simulink model "accumulator_basic_ok"  (R2019b)
settings: Solver=ode4  StartTime=0.0  StopTime=100  FixedStep=0.001  RelTol=1e-3
values from neighbouring files (symbols this model uses):
  Am = 7.2    [value.m]
  Aw = 3.812*10^(-12)    (= 3.812e-12)    [value.m]
  valve_radius = 0.01    [value.m]
undefined symbols (not defined in the file or in its folder): sigbuilder_block
libraries: fl_lib x11, nesl_utility x8, sh_lib x5
settings Model: Creator=remil  LastModifiedBy=remil
settings SimscapeCC: SimscapeLogType=all  SimscapeLogSimulationStatistics=on  SimscapeLogOpenViewer=on

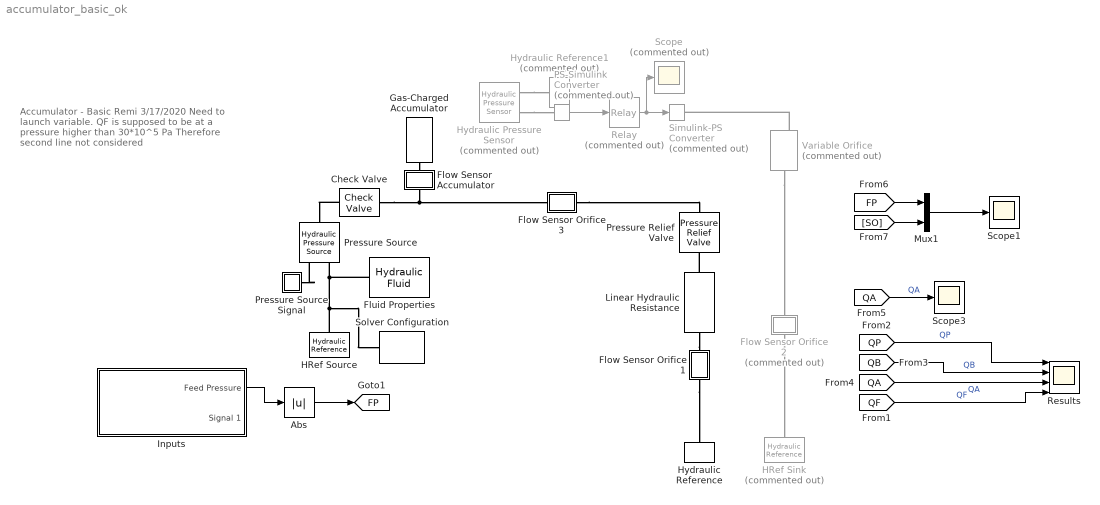
== system accumulator_basic_ok ==
  note: Accumulator - Basic
      | Remi 3/17/2020
      | Need to launch variable.
      | QF is supposed to be at a pressure
      | higher than 30*10^5 Pa Therefore
      | second line not considered
  Abs : Abs
  Check Valve : sh_lib/Valves/Directional Valves/Check Valve  Tag=Factory Generic  area_max=pi*(valve_radius)^2 m^2  pres_crack=30000 Pa  pres_max=120000 Pa  C_d=0.7  A_leak=1e-12 m^2  lam_spec=1  B_lam=0.999  Re_cr=12  dynamic=1  tau=0.1 s  area_init=1e-12 m^2
      settings: SourceProductName=Simscape Fluids  SourceProductBaseCode=SH  InternalSimscapePortConfiguration="{\"Bottom\":[],\"Left\":[{\"id\":\"A\",\"label\":\"A\",\"type\":\"foundation.hydraulic.hydraulic\"}],\"Right\":[{\"id\":\"B\",\"label\":\"B\",\"type\":\"foundation.hydraulic.hydraulic\"}],\"Top\":[]}"
  Flow Sensor Accumulator : Subsystem
      mask Display: disp('QA')
  Flow Sensor Orifice 1 : Subsystem
      mask Display: disp('QP');
  Flow Sensor Orifice 2 : Subsystem  Commented=on
      mask Display: disp('QB');
  Flow Sensor Orifice 3 : Subsystem
      mask Display: disp('QF');
  Fluid Properties : sh_lib/Hydraulic Utilities/Hydraulic Fluid  DataSource=1  SelFluid=1  SysTemp=60  TrapAir=0.005  ViscDerFactor=1  range_error=2
      settings: SourceProductName=Simscape Fluids
  Gas-Charged Accumulator : sh_lib/Accumulators/Gas-Charged Accumulator  capacity=2.5 gal  dead_volume=0.08 l  pr_preload=30e5 Pa  k_sh=1.4  stiff_coeff=1e12 Pa/m^3  penetr_coeff=1e10 s*Pa/m^6  flow_rate_specify=off  flow_rate_priority=High  flow_rate=0.005 m^3/s  flow_rate_nominal_specify=off  flow_rate_nominal_unit=m^3/s  flow_rate_nominal_value=1  liquid_volume_specify=on  liquid_volume_priority=High  liquid_volume=0 gal  liquid_volume_nominal_specify=off  liquid_volume_nominal_unit=m^3  liquid_volume_nominal_value=1  liquid_pressure_specify=off  liquid_pressure_priority=None  liquid_pressure=1.01325e+5 Pa  liquid_pressure_nominal_specify=off  liquid_pressure_nominal_unit=Pa  liquid_pressure_nominal_value=1
      settings: SourceProductName=Simscape Fluids  SourceProductBaseCode=SH  InternalSimscapePortConfiguration="{\"Bottom\":[],\"Left\":[],\"Right\":[{\"id\":\"A\",\"label\":\"A\",\"type\":\"foundation.hydraulic.hydraulic\"}],\"Top\":[]}"
  HRef Sink : fl_lib/Hydraulic/Hydraulic Elements/Hydraulic Reference  Tag=Factory Generic  Commented=on
      settings: SourceProductName=Simscape
  HRef Source : fl_lib/Hydraulic/Hydraulic Elements/Hydraulic Reference  Tag=Factory Generic
      settings: SourceProductName=Simscape
  Hydraulic Pressure Sensor : fl_lib/Hydraulic/Hydraulic Sensors/Hydraulic Pressure Sensor  Commented=on
      settings: SourceProductName=Simscape
  Hydraulic Reference : fl_lib/Hydraulic/Hydraulic Elements/Hydraulic Reference
      settings: SourceProductName=Simscape
  Hydraulic Reference1 : fl_lib/Hydraulic/Hydraulic Elements/Hydraulic Reference  Commented=on
      settings: SourceProductName=Simscape
  "Inputs " : Subsystem  Tag=STV Subsys  LoadFcn=sigbuilder_block('load');  StartFcn=sigbuilder_block('start');  StopFcn=sigbuilder_block('stop');  ClipboardFcn=sigbuilder_block('clipboard');  mask(Sigbuilder block){tuvar=[0:10]}
      mask help: Sigbuilder GUI
      mask init:
      | if ~strcmp(get_param(bdroot(gcbh),'SimulationStatus'),'stopped') tuvar = sigbuilder_block('maskInit'); end
      settings: CopyFcn=sigbuilder_block('copy');  DeleteFcn=sigbuilder_block('delete');  ModelCloseFcn=sigbuilder_block('modelClose');  PreSaveFcn=sigbuilder_block('preSave');  PauseFcn=sigbuilder_block('pause')  ContinueFcn=sigbuilder_block('continue')  NameChangeFcn=sigbuilder_block('namechange');  OpenFcn=sigbuilder_block('open',[6 30 1428 681.75 ]);  CloseFcn=sigbuilder_block('close');
      mask Display: plot(0, 0, 100, 100,[2, 2, 32, 32, 2], [68, 8, 8, 68, 68],[32, 2], [38, 38], [32, 19, 2],[53, 60, 44], [32, 17, 17, 2],[16, 16, 31, 31]);txt = getActiveGroup(gcbh);text(2, 100, txt,'verticalAlignment', 'top');
  Linear Hydraulic Resistance : fl_lib/Hydraulic/Hydraulic Elements/Linear Hydraulic Resistance  resistance=1/(Am*Aw) Pa/(m^3/s)  q_specify=off  q_priority=None  q=0.001 m^3/s  q_nominal_specify=off  q_nominal_unit=m^3/s  q_nominal_value=1  p_specify=off  p_priority=None  p=0 Pa  p_nominal_specify=off  p_nominal_unit=Pa  p_nominal_value=1
      settings: SourceProductName=Simscape  SourceProductBaseCode=SS  InternalSimscapePortConfiguration="{\"Bottom\":[],\"Left\":[{\"id\":\"A\",\"label\":\"A\",\"type\":\"foundation.hydraulic.hydraulic\"}],\"Right\":[{\"id\":\"B\",\"label\":\"B\",\"type\":\"foundation.hydraulic.hydraulic\"}],\"Top\":[]}"
  Mux1 : Mux  Inputs=2
      settings: DisplayOption=signals
  PS-Simulink Converter : nesl_utility/PS-Simulink Converter  Commented=on  PhysicalDomain=network_engine_domain  SubClassName=ps_output  LeftPortType=input  RightPortType=output  PseudoPeriodic=off  Frequencies=[]  Unit=inherit  AffineConversion=off
  Pressure Source : fl_lib/Hydraulic/Hydraulic Sources/Hydraulic Pressure Source  Tag=Factory Generic
      settings: SourceProductName=Simscape  SourceProductBaseCode=SS  InternalSimscapePortConfiguration="{\"Bottom\":[],\"Left\":[{\"id\":\"P\",\"label\":\"P\",\"type\":\"foundation.hydraulic.hydraulic\"}],\"Right\":[{\"id\":\"S\",\"label\":\"S\",\"type\":\"input\"},{\"id\":\"T\",\"label\":\"T\",\"type\":\"foundation.hydraulic.hydraulic\"}],\"Top\":[]}"
  Pressure Source Signal : Subsystem
      mask Display: disp('FP')
  Pressure Relief Valve : sh_lib/Valves/Pressure Control Valves/Pressure Relief Valve  valve_area_spec=1  p_diff_TLU=[30.15e5 : 15e3 : 31.35e5] Pa  area_TLU=[1 : 1 : 9] .* 1e-5 m^2  area_max=pi*(valve_radius)^2 m^2  pres_set=30e5 Pa  reg_range=5e5 Pa  C_d=0.7  A_leak=1e-12 m^2  lam_spec=1  B_lam=0.999  Re_cr=12  dynamic=0  tau=0.1 s  area_init=1e-12 m^2
      settings: SourceProductName=Simscape Fluids  SourceProductBaseCode=SH  InternalSimscapePortConfiguration="{\"Bottom\":[],\"Left\":[{\"id\":\"A\",\"label\":\"A\",\"type\":\"foundation.hydraulic.hydraulic\"}],\"Right\":[{\"id\":\"B\",\"label\":\"B\",\"type\":\"foundation.hydraulic.hydraulic\"}],\"Top\":[]}"
  Relay : Relay  Commented=on  OnSwitchValue=30*10^5  OffSwitchValue=30*10^5  OnOutputValue=0  OffOutputValue=0.01
  Results : Scope  NumInputPorts=4
  Scope : Scope  Commented=on
  Scope1 : Scope
  Scope3 : Scope
  Simulink-PS Converter : nesl_utility/Simulink-PS Converter  Commented=on  PhysicalDomain=network_engine_domain  SubClassName=ps_input  LeftPortType=input  RightPortType=output  PseudoPeriodic=off  Frequencies=[]  NoiseDistribution=none  NoiseParameters=[]  Unit=1  AffineConversion=off  FilteringAndDerivatives=filter  SimscapeFilterOrder=1  InputFilterTimeConstant=0.001  UdotUserProvided=0
  Solver Configuration : nesl_utility/Solver Configuration  PhysicalDomain=network_engine_domain  SubClassName=solver  LeftPortType=input  RightPortType=generic  Tones=[]  Harmonics=[]  SimulateNoise=off  Profile=off  UseLocalSampling=off  EnableSwitchedLinearOptims=on  FrequencyDomain=off  UseCCode=off  RelTol=0.001  AbsTol=1e-06  MinStep=1e-09  ToWorkspace=off  RevertToSquareIcSolve=off  NumHomotopyIterations=100  PhasorMode=off  PhasorModeNumHarmonics=1  DoDC=on  ResidualTolerance=1e-9  UseLocalSolver=on  LocalSolverChoice=NE_BACKWARD_EULER_ADVANCER  LocalSolverSampleTime=.001  DoFixedCost=on  MaxNonlinIter=3  MaxModeIter=2  LinearAlgebra=auto  EquationFormulation=NE_TIME_EF  DelaysMemoryBudget=1024  AutomaticFiltering=on  FilteringTimeConstant=0.001  PartitionStorageMethod=AS_NEEDED  PartitionMemoryBudget=1024  PartitionMethod=FAST
  Variable Orifice : sh_lib/Orifices/Variable Orifice  Commented=on  mdl_type=1  area_max=pi*(valve_radius)^2 m^2  opening_max=2*0.01 m  opening_tab=[-.002, 0, .002, .005, .015] m  area_tab=[1e-09, 2.0352e-07, 4.0736e-05, .00011438, .00034356] m^2  pressure_tab=[-10000000, -5000000, -2000000, 2000000, 5000000, 10000000] Pa  flow_rate_tab=[-1e-07, -7.0711e-08, -4.4721e-08, 4.4721e-08, 7.0711e-08, 1e-07; -2.0352e-05, -1.4391e-05, -9.1017e-06, 9.1017e-06, 1.4391e-05, 2.0352e-05; -.0040736, -.0028805, -.0018218, .0018218, .0028805, .0040736; -.011438, -.0080879, -.0051152, .0051152, .0080879, .011438; -.034356, -.024293, -.015364, .015364, .024293, .034356] m^3/s  interp_method=1  extrap_method=1  or=1  C_d=0.7  x_0=0 m  A_leak=1e-12 m^2  lam_spec=1  B_lam=0.999  Re_cr=12  flow_rate_specify=on  flow_rate_priority=High  flow_rate=0 m^3/s  flow_rate_nominal_specify=off  flow_rate_nominal_unit=m^3/s  flow_rate_nominal_value=1  pressure_drop_specify=off  pressure_drop_priority=None  pressure_drop=0 Pa  pressure_drop_nominal_specify=off  pressure_drop_nominal_unit=Pa  pressure_drop_nominal_value=1
      settings: SourceProductName=Simscape Fluids  SourceProductBaseCode=SH  InternalSimscapePortConfiguration="{\"Bottom\":[],\"Left\":[{\"id\":\"S\",\"label\":\"S\",\"type\":\"input\"},{\"id\":\"A\",\"label\":\"A\",\"type\":\"foundation.hydraulic.hydraulic\"}],\"Right\":[{\"id\":\"B\",\"label\":\"B\",\"type\":\"foundation.hydraulic.hydraulic\"}],\"Top\":[]}"
  tag scope: FP=global
  wires:
  Abs/1 -> [FP]
  [QP] -> Results/1  "QP"
  [QB] -> Results/2  "QB"
  [QA] -> Results/3  "QA"
  [QA] -> Scope3/1  "QA"
  PS-Simulink Converter/1 -> Relay/1
  Relay/1 -> Scope/1, Simulink-PS Converter/1
  Mux1/1 -> Scope1/1
  [FP] -> Mux1/1
  [SO] -> Mux1/2
  [QF] -> Results/4  "QF"
  "Inputs "/1(Feed Pressure) -> Abs/1
  connections:
  Flow Sensor Orifice 2/LConn1 -- HRef Sink/LConn1
  Pressure Source/RConn2 -- Solver Configuration/RConn1 -- HRef Source/LConn1 -- Fluid Properties/RConn1
  Gas-Charged Accumulator/RConn1 -- Flow Sensor Accumulator/RConn1
  Pressure Source Signal/RConn1 -- Pressure Source/RConn1
  Variable Orifice/LConn1 -- Simulink-PS Converter/RConn1
  Flow Sensor Orifice 3/RConn1 -- Pressure Relief Valve/LConn1
  Check Valve/RConn1 -- Flow Sensor Accumulator/LConn1 -- Flow Sensor Orifice 3/LConn1
  Hydraulic Pressure Sensor/RConn2 -- PS-Simulink Converter/LConn1
  Hydraulic Pressure Sensor/RConn1 -- Hydraulic Reference1/LConn1
  Linear Hydraulic Resistance/RConn1 -- Flow Sensor Orifice 1/LConn1
  Flow Sensor Orifice 1/RConn1 -- Hydraulic Reference/LConn1
  Check Valve/LConn1 -- Pressure Source/LConn1
  Linear Hydraulic Resistance/LConn1 -- Pressure Relief Valve/RConn1
  Variable Orifice/RConn1 -- Flow Sensor Orifice 2/RConn1

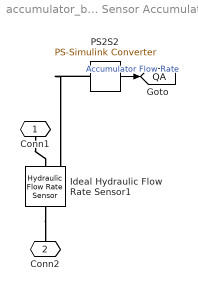
== system accumulator_basic_ok/Flow Sensor Accumulator ==
  Ideal Hydraulic Flow Rate Sensor1 : fl_lib/Hydraulic/Hydraulic Sensors/Hydraulic Flow Rate Sensor  Tag=Factory Generic
      settings: SourceProductName=Simscape
  PS2S2 : nesl_utility/PS-Simulink Converter  PhysicalDomain=network_engine_domain  SubClassName=ps_output  LeftPortType=input  RightPortType=output  PseudoPeriodic=off  Frequencies=[]  Unit=1  AffineConversion=off
  Conn1 : PMIOPort  Side=Right
  Conn2 : PMIOPort  Port=2  Side=Left
  tag scope: QA=global
  wires:
  PS2S2/1 -> [QA]  "Accumulator Flow Rate"
  connections:
  PS2S2/LConn1 -- Ideal Hydraulic Flow Rate Sensor1/RConn1
  Conn1/RConn1 -- Ideal Hydraulic Flow Rate Sensor1/RConn2
  Ideal Hydraulic Flow Rate Sensor1/LConn1 -- Conn2/RConn1

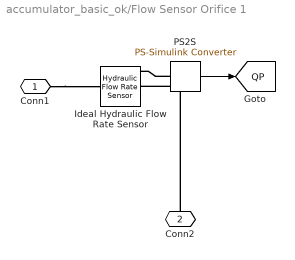
== system accumulator_basic_ok/Flow Sensor Orifice 1 ==
  Ideal Hydraulic Flow Rate Sensor : fl_lib/Hydraulic/Hydraulic Sensors/Hydraulic Flow Rate Sensor  Tag=Factory Generic
      settings: SourceProductName=Simscape
  PS2S : nesl_utility/PS-Simulink Converter  PhysicalDomain=network_engine_domain  SubClassName=ps_output  LeftPortType=input  RightPortType=output  PseudoPeriodic=off  Frequencies=[]  Unit=1  AffineConversion=off
  Conn1 : PMIOPort  Side=Left
  Conn2 : PMIOPort  Port=2  Side=Right
  tag scope: QP=global
  wires:
  PS2S/1 -> [QP]
  connections:
  PS2S/LConn1 -- Ideal Hydraulic Flow Rate Sensor/RConn1
  Conn2/RConn1 -- Ideal Hydraulic Flow Rate Sensor/RConn2
  Conn1/RConn1 -- Ideal Hydraulic Flow Rate Sensor/LConn1

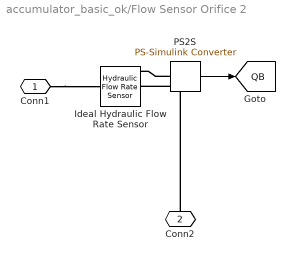
== system accumulator_basic_ok/Flow Sensor Orifice 2 ==
  Ideal Hydraulic Flow Rate Sensor : fl_lib/Hydraulic/Hydraulic Sensors/Hydraulic Flow Rate Sensor  Tag=Factory Generic
      settings: SourceProductName=Simscape
  PS2S : nesl_utility/PS-Simulink Converter  PhysicalDomain=network_engine_domain  SubClassName=ps_output  LeftPortType=input  RightPortType=output  PseudoPeriodic=off  Frequencies=[]  Unit=1  AffineConversion=off
  Conn1 : PMIOPort  Side=Left
  Conn2 : PMIOPort  Port=2  Side=Right
  tag scope: QB=global
  wires:
  PS2S/1 -> [QB]
  connections:
  PS2S/LConn1 -- Ideal Hydraulic Flow Rate Sensor/RConn1
  Conn2/RConn1 -- Ideal Hydraulic Flow Rate Sensor/RConn2
  Conn1/RConn1 -- Ideal Hydraulic Flow Rate Sensor/LConn1

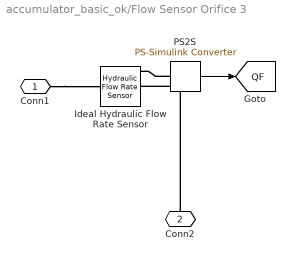
== system accumulator_basic_ok/Flow Sensor Orifice 3 ==
  Ideal Hydraulic Flow Rate Sensor : fl_lib/Hydraulic/Hydraulic Sensors/Hydraulic Flow Rate Sensor  Tag=Factory Generic
      settings: SourceProductName=Simscape
  PS2S : nesl_utility/PS-Simulink Converter  PhysicalDomain=network_engine_domain  SubClassName=ps_output  LeftPortType=input  RightPortType=output  PseudoPeriodic=off  Frequencies=[]  Unit=1  AffineConversion=off
  Conn1 : PMIOPort  Side=Left
  Conn2 : PMIOPort  Port=2  Side=Right
  tag scope: QF=global
  wires:
  PS2S/1 -> [QF]
  connections:
  PS2S/LConn1 -- Ideal Hydraulic Flow Rate Sensor/RConn1
  Conn2/RConn1 -- Ideal Hydraulic Flow Rate Sensor/RConn2
  Conn1/RConn1 -- Ideal Hydraulic Flow Rate Sensor/LConn1

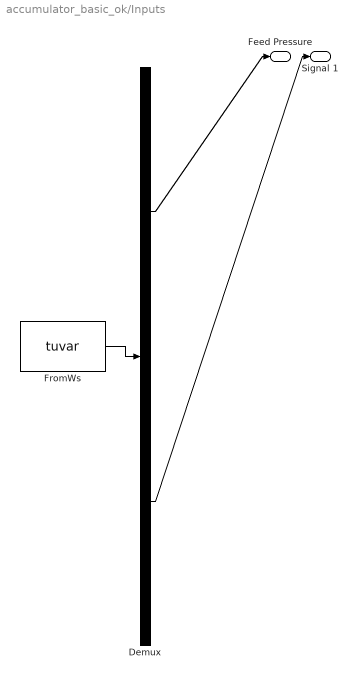
== system accumulator_basic_ok/Inputs  ==
  Demux : Demux  Tag=STV Demux  Outputs=2
  FromWs : FromWorkspace  Tag=STV FromWs  VariableName=tuvar  SampleTime=0
      SigBuilderData=|
      | common.afterFinalStr = 'Extrapolate'
      | common.sampleTime = 0
      | dataSet.timeRange = [0 100]
      | dataSet.name = 'Group 1'
      | sbobj.Groups.Name = 'Group 1'
      | sbobj.Groups.Signals(1).Name = 'Feed Pressure'
      | sbobj.Groups.Signals(1).XData = [0 0.142857142857 0.285714285714 0.428571428571 0.571428571429 0.714285714286 0.857142857143 1 1.14285714286 1.28571428571 1.42857142857 1.57142857143 ... (701 elements, 1x701)]
      | sbobj.Groups.Signals(1).YData = [1 639386.808423 1268273.91955 1876336.0244 2453588.76002 2990553.65246 3478413.75302 3909158.41234 4275714.81503 4572064.11508 4793340.26518 4935909.91707 ... (701 elements, 1x701)]
      | sbobj.Groups.Signals(2).Name = 'Signal 1'
      | sbobj.Groups.Signals(2).XData = [0 100]
      | sbobj.Groups.Signals(2).YData = [3500000 3500000]
      | sbobj.Groups.TimeRange = [0 100]
  Feed Pressure : Outport  Tag=STV Outport
  Signal 1 : Outport  Tag=STV Outport  Port=2
  wires:
  FromWs/1 -> Demux/1
  Demux/1 -> Feed Pressure/1
  Demux/2 -> Signal 1/1

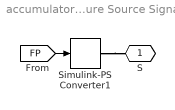
== system accumulator_basic_ok/Pressure Source Signal ==
  Simulink-PS Converter1 : nesl_utility/Simulink-PS Converter  PhysicalDomain=network_engine_domain  SubClassName=ps_input  LeftPortType=input  RightPortType=output  PseudoPeriodic=off  Frequencies=[]  NoiseDistribution=none  NoiseParameters=[]  Unit=1  AffineConversion=off  FilteringAndDerivatives=filter  SimscapeFilterOrder=1  InputFilterTimeConstant=.001  UdotUserProvided=0
  S : PMIOPort  Side=Right
  wires:
  [FP] -> Simulink-PS Converter1/1
  connections:
  Simulink-PS Converter1/RConn1 -- S/RConn1
